simulink model "Commande_1_ModeGlissant"  (R2015a)
settings: Solver=ode45  StartTime=0.0  StopTime=5  RelTol=1e-3
undefined symbols (not defined in the file or in its folder): sfun3d
(part 1 of 2)
settings Model: Creator=user  LastModifiedBy=user

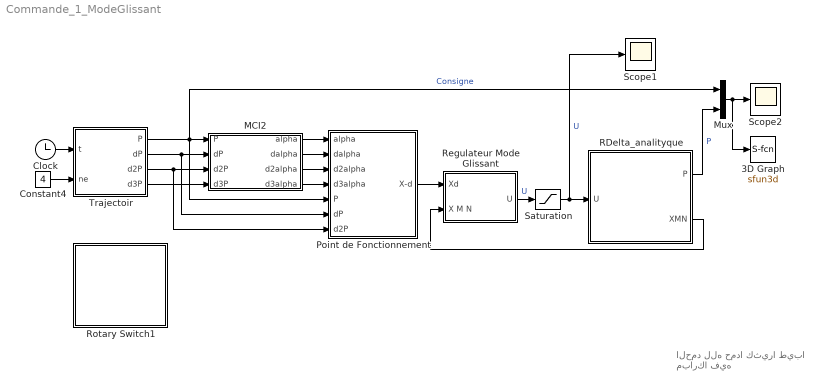
== system Commande_1_ModeGlissant ==
  note: الحمد لله حمدا كثيرا طيبا مباركا فيه
  3D Graph : S-Function  LoadFcn=sfun3d([],[],[],'LoadBlock')  StartFcn=sfun3d([],[],[],'Start')  StopFcn=sfun3d([],[],[],'Stop')  FunctionName=sfun3d  Parameters=ax,T,np,cp,gd,ls,mk  mask(3D Graph){np=2, ax=[-1 1 -1 1 -2 0]*0.3, cp=[3 2 1], gd=on, ls=-, mk=none, T=0.0001}
      mask prompts: np "Number of point (lines)"; ax "[xmin xmax  ymin ymax zmin zmax]"; cp "Camera position (use [0 0 1] for 2D XY view)"; gd "Grid (on|off)"; ls "LineStyle"; mk "Marker"; T "Sampling Time"
      mask help:
      | This block plots the position of several points in the XYZ space. The input contains the coordinates of all the points (x1,y1,z1,x2,y2,z2,...).
      | The number of points (lines), the XYZ ranges, camera position, grid, linestyle, marker and sampling time, can be set as mask parameters.
      settings: CopyFcn=sfun3d([],[],[],'CopyBlock')  DeleteFcn=sfun3d([],[],[],'DeleteBlock')  NameChangeFcn=sfun3d([],[],[],'NameChange')
      mask Help:
      | This block plots the position of several points in the XYZ space. The input contains the coordinates of all the points (x1,y1,z1,x2,y2,z2,...).
      | The number of points (lines), the XYZ ranges, camera position, grid, linestyle, marker and sampling time, can be set as mask parameters.
      mask TypeOptions ls: - | -- | : | -. | none
      mask TypeOptions mk: none | . | + | o | * | x | square | diamond | v | ^ | > | < | pentagram | hexagram
      mask Display: plot([.05 .95 .95 .05 .05],[.45 .45 .95 .95 .45], 0.5+cos(0:0.1:2*pi)*0.3,0.7+sin(0:0.1:2*pi)*0.2)
  Clock : Clock
  Constant4 : Constant  Value=4
  MCI2 : MATLAB Function  TreatAsAtomicUnit=on
  Mux : Mux  Inputs=2
  Point de Fonctionnement : Subsystem
  RDelta_analityque : Subsystem
      mask Display:
      | image(imread('DeltaImage2.PNG'))
      | 
      | port_label('input',1,'U')
      | 
      | port_label('output',1,'P')
      | 
      | port_label('output',2,'XMN')
  Regulateur Mode Glissant : Subsystem
  Rotary Switch1 : Subsystem  DialogController=hmiCreateDDGDialog  IsWebBlock=on  mask(MathWorksWebBlock){webBlockId=84b08da5-f823-455a-b5c0-7d4cf8879998, webBlockType=discreteknob, ShowInLibBrowser=on, ShowInitialText=on, HMISrcModelName=Commande_1_ModeGlissant}
      mask prompts: webBlockId "WebBlock Id"; webBlockType "WebBlock Type"; HMISrcModelName "Source Model"
      mask Help: helpview([docroot '/mapfiles/simulink.map'], 'hmi_rotary_switch')
      mask Display:
      | model = bdroot(gcb);
      | if strcmp(get_param(model,'BlockDiagramType'), 'library')
      |     image([(matlabroot) '/toolbox/simulink/hmi/icons/DiscreteKnob.png']);
      | end
  Saturation : Saturate  UpperLimit=24  LowerLimit=-24
  Scope1 : Scope
      settings: YMax=4.5
  Scope2 : Scope
      settings: YMin=-0.325  YMax=0.225
  Trajectoir : MATLAB Function  TreatAsAtomicUnit=on
  wires:
  RDelta_analityque/1(P) -> Mux/2  "P"
  Trajectoir/1(P) -> Point de Fonctionnement/5(P), Mux/1, MCI2/1(P)  "Consigne"
  Trajectoir/2(dP) -> Point de Fonctionnement/6(dP), MCI2/2(dP)
  Trajectoir/3(d2P) -> Point de Fonctionnement/7(d2P), MCI2/3(d2P)
  MCI2/3(d2alpha) -> Point de Fonctionnement/3(d2alpha)
  MCI2/2(dalpha) -> Point de Fonctionnement/2(dalpha)
  Clock/1 -> Trajectoir/1(t)
  Constant4/1 -> Trajectoir/2(ne)
  MCI2/1(alpha) -> Point de Fonctionnement/1(alpha)
  MCI2/4(d3alpha) -> Point de Fonctionnement/4(d3alpha)
  Trajectoir/4(d3P) -> MCI2/4(d3P)
  Mux/1 -> Scope2/1, 3D Graph/1
  Point de Fonctionnement/1(X-d) -> Regulateur Mode Glissant/1(Xd)
  RDelta_analityque/2(XMN) -> Regulateur Mode Glissant/2(X M N)
  Saturation/1 -> Scope1/1, RDelta_analityque/1(U)  "U"
  Regulateur Mode Glissant/1(U) -> Saturation/1  "U"

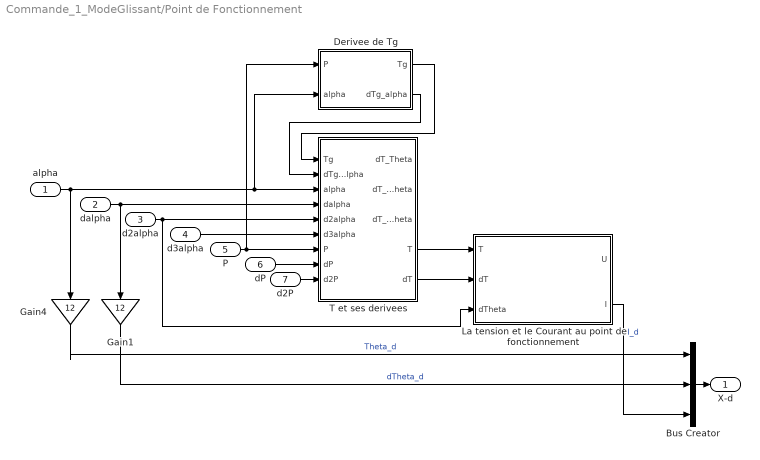
== system Commande_1_ModeGlissant/Point de Fonctionnement ==
  alpha : Inport
  dalpha : Inport  Port=2
  d2alpha : Inport  Port=3
  d3alpha : Inport  Port=4
  P : Inport  Port=5
  dP : Inport  Port=6
  d2P : Inport  Port=7
  Bus Creator : BusCreator  Inputs=3
  Derivee de Tg : Subsystem
  Gain1 : Gain  Gain=12
  Gain4 : Gain  Gain=12
  La tension et le Courant au point de fonctionnement : MATLAB Function  TreatAsAtomicUnit=on
  T et ses derivees : Subsystem
  X-d : Outport
  wires:
  alpha/1 -> Derivee de Tg/2(alpha), T et ses derivees/3(alpha), Gain4/1
  dalpha/1 -> Gain1/1, T et ses derivees/4(dalpha)
  P/1 -> Derivee de Tg/1(P), T et ses derivees/7(P)
  dP/1 -> T et ses derivees/8(dP)
  d2P/1 -> T et ses derivees/9(d2P)
  T et ses derivees/5(dT) -> La tension et le Courant au point de fonctionnement/2(dT)
  Derivee de Tg/2(dTg_alpha) -> T et ses derivees/2(dTg_alpha)
  Derivee de Tg/1(Tg) -> T et ses derivees/1(Tg)
  d3alpha/1 -> T et ses derivees/6(d3alpha)
  T et ses derivees/4(T) -> La tension et le Courant au point de fonctionnement/1(T)
  Bus Creator/1 -> X-d/1
  Gain4/1 -> Bus Creator/1  "Theta_d"
  Gain1/1 -> Bus Creator/2  "dTheta_d"
  d2alpha/1 -> La tension et le Courant au point de fonctionnement/3(dTheta), T et ses derivees/5(d2alpha)
  La tension et le Courant au point de fonctionnement/2(I) -> Bus Creator/3  "I_d"

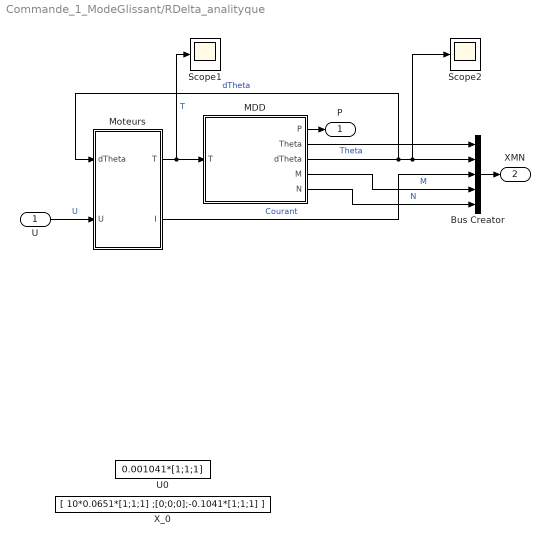
== system Commande_1_ModeGlissant/RDelta_analityque ==
  U : Inport
  Bus Creator : BusCreator  Inputs=5
  MDD : Subsystem
      mask Display:
      | image(imread('DeltaImage2.PNG'))
      | port_label('input',1,'T')
      | port_label('output',1,'P')
      | port_label('output',2,'Theta')
      | port_label('output',3,'dTheta')
      | port_label('output',4,'M')
      | port_label('output',5,'N')
  Moteurs : Subsystem
      mask Display:
      | image('image_motor.jpg')
      | port_label('output',1,'T')
      | port_label('output',2,'I')
      | port_label('input',1,'U')
      | port_label('input',2,'dTheta')
  Scope1 : Scope
      settings: YMin=-0.2  YMax=0.175  SaveName=ScopeData3
  Scope2 : Scope
      settings: YMin=0.774525  YMax=0.774531  SaveName=ScopeData7
  U0 : Constant  Value=0.001041*[1;1;1]
  X_0 : Constant  Value=[ 10*0.0651*[1;1;1] ;[0;0;0];-0.1041*[1;1;1] ]
  P : Outport
  XMN : Outport  Port=2
  wires:
  Moteurs/2(I) -> Bus Creator/3  "Courant"
  U/1 -> Moteurs/2(U)  "U"
  MDD/2(Theta) -> Bus Creator/1  "Theta"
  MDD/3(dTheta) -> Moteurs/1(dTheta), Bus Creator/2, Scope2/1  "dTheta"
  Moteurs/1(T) -> Scope1/1, MDD/1(T)  "T"
  MDD/1(P) -> P/1
  MDD/4(M) -> Bus Creator/4  "M"
  MDD/5(N) -> Bus Creator/5  "N"
  Bus Creator/1 -> XMN/1

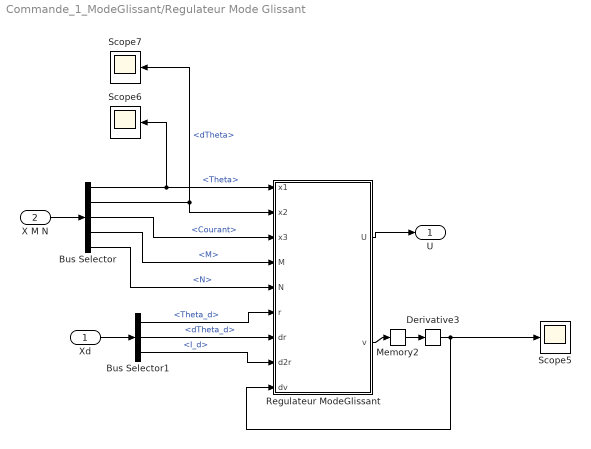
== system Commande_1_ModeGlissant/Regulateur Mode Glissant ==
  Xd : Inport
  X M N : Inport  Port=2
  Bus Selector : BusSelector  OutputSignals=Theta,dTheta,Courant,M,N
  Bus Selector1 : BusSelector  OutputSignals=Theta_d,dTheta_d,I_d
  Derivative3 : Derivative
  Memory2 : Memory  X0=[0;0;0]
  Regulateur ModeGlissant : MATLAB Function  TreatAsAtomicUnit=on
  Scope5 : Scope
      settings: YMin=-2000  YMax=18000  SaveName=ScopeData6
  Scope6 : Scope
      settings: YMin=-2000  YMax=18000  SaveName=ScopeData9
  Scope7 : Scope
      settings: YMin=-2000  YMax=18000  SaveName=ScopeData10
  U : Outport
  wires:
  Regulateur ModeGlissant/1(U) -> U/1
  Bus Selector/1 -> Scope6/1, Regulateur ModeGlissant/1(x1)  "<Theta>"
  Bus Selector/2 -> Scope7/1, Regulateur ModeGlissant/2(x2)  "<dTheta>"
  Bus Selector/3 -> Regulateur ModeGlissant/3(x3)  "<Courant>"
  Bus Selector/4 -> Regulateur ModeGlissant/4(M)  "<M>"
  Bus Selector/5 -> Regulateur ModeGlissant/5(N)  "<N>"
  X M N/1 -> Bus Selector/1
  Xd/1 -> Bus Selector1/1
  Regulateur ModeGlissant/2(v) -> Memory2/1
  Memory2/1 -> Derivative3/1
  Derivative3/1 -> Regulateur ModeGlissant/9(dv), Scope5/1
  Bus Selector1/1 -> Regulateur ModeGlissant/6(r)  "<Theta_d>"
  Bus Selector1/2 -> Regulateur ModeGlissant/7(dr)  "<dTheta_d>"
  Bus Selector1/3 -> Regulateur ModeGlissant/8(d2r)  "<I_d>"

== system Commande_1_ModeGlissant/Rotary Switch1 ==

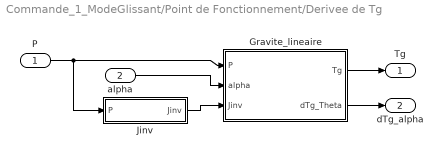
== system Commande_1_ModeGlissant/Point de Fonctionnement/Derivee de Tg ==
  P : Inport
  alpha : Inport  Port=2
  Gravite_lineaire : MATLAB Function  TreatAsAtomicUnit=on
  Jinv : MATLAB Function  TreatAsAtomicUnit=on
  Tg : Outport
  dTg_alpha : Outport  Port=2
  wires:
  P/1 -> Jinv/1(P), Gravite_lineaire/1(P)
  alpha/1 -> Gravite_lineaire/2(alpha)
  Jinv/1(Jinv) -> Gravite_lineaire/3(Jinv)
  Gravite_lineaire/2(dTg_Theta) -> dTg_alpha/1
  Gravite_lineaire/1(Tg) -> Tg/1

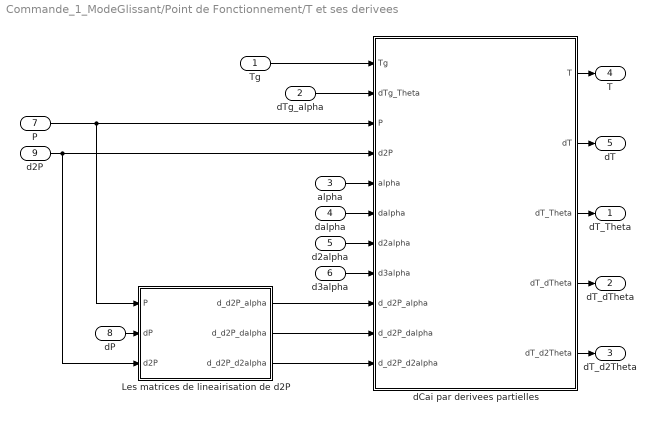
== system Commande_1_ModeGlissant/Point de Fonctionnement/T et ses derivees ==
  Tg : Inport
  dTg_alpha : Inport  Port=2
  alpha : Inport  Port=3
  dalpha : Inport  Port=4
  d2alpha : Inport  Port=5
  d3alpha : Inport  Port=6
  P : Inport  Port=7
  dP : Inport  Port=8
  d2P : Inport  Port=9
  "Les matrices de lineairisation de d2P  " : MATLAB Function  TreatAsAtomicUnit=on
  "dCai par derivees partielles " : MATLAB Function  TreatAsAtomicUnit=on
  dT_Theta : Outport
  dT_dTheta : Outport  Port=2
  dT_d2Theta : Outport  Port=3
  T : Outport  Port=4
  dT : Outport  Port=5
  wires:
  "Les matrices de lineairisation de d2P  "/2(d_d2P_dalpha) -> "dCai par derivees partielles "/10(d_d2P_dalpha)
  "Les matrices de lineairisation de d2P  "/3(d_d2P_d2alpha) -> "dCai par derivees partielles "/11(d_d2P_d2alpha)
  "Les matrices de lineairisation de d2P  "/1(d_d2P_alpha) -> "dCai par derivees partielles "/9(d_d2P_alpha)
  P/1 -> "Les matrices de lineairisation de d2P  "/1(P), "dCai par derivees partielles "/3(P)
  d2P/1 -> "Les matrices de lineairisation de d2P  "/3(d2P), "dCai par derivees partielles "/4(d2P)
  alpha/1 -> "dCai par derivees partielles "/5(alpha)
  dalpha/1 -> "dCai par derivees partielles "/6(dalpha)
  d2alpha/1 -> "dCai par derivees partielles "/7(d2alpha)
  dP/1 -> "Les matrices de lineairisation de d2P  "/2(dP)
  "dCai par derivees partielles "/3(dT_Theta) -> dT_Theta/1
  "dCai par derivees partielles "/4(dT_dTheta) -> dT_dTheta/1
  "dCai par derivees partielles "/5(dT_d2Theta) -> dT_d2Theta/1
  dTg_alpha/1 -> "dCai par derivees partielles "/2(dTg_Theta)
  Tg/1 -> "dCai par derivees partielles "/1(Tg)
  d3alpha/1 -> "dCai par derivees partielles "/8(d3alpha)
  "dCai par derivees partielles "/1(T) -> T/1
  "dCai par derivees partielles "/2(dT) -> dT/1

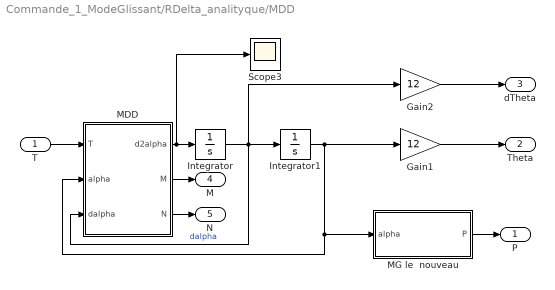
== system Commande_1_ModeGlissant/RDelta_analityque/MDD ==
  T : Inport
  Gain1 : Gain  Gain=12
  Gain2 : Gain  Gain=12
  Integrator : Integrator  InitialCondition=[0;0;0]
  Integrator1 : Integrator  InitialCondition=0.0651*[1;1;1]
  MDD : Subsystem
  MG le  nouveau : MATLAB Function  TreatAsAtomicUnit=on
  Scope3 : Scope
      settings: TimeRange=2.077341948455237  YMin=0.00075  YMax=0.00275  SaveName=ScopeData2
  P : Outport
  Theta : Outport  Port=2
  dTheta : Outport  Port=3
  M : Outport  Port=4
  N : Outport  Port=5
  wires:
  MDD/1(d2alpha) -> Scope3/1, Integrator/1
  Integrator/1 -> Gain2/1, MDD/3(dalpha), Integrator1/1  "dalpha"
  Integrator1/1 -> MG le  nouveau/1(alpha), MDD/2(alpha), Gain1/1
  T/1 -> MDD/1(T)
  MG le  nouveau/1(P) -> P/1
  Gain1/1 -> Theta/1
  Gain2/1 -> dTheta/1
  MDD/2(M) -> M/1
  MDD/3(N) -> N/1

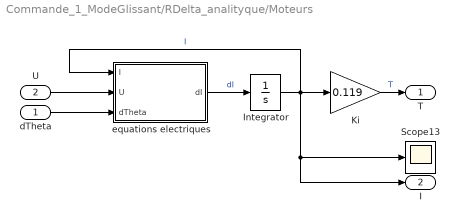
== system Commande_1_ModeGlissant/RDelta_analityque/Moteurs ==
  dTheta : Inport
  U : Inport  Port=2
  Integrator : Integrator  InitialCondition=-0.105*[1;1;1]
  Ki : Gain  Gain=0.119
  Scope13 : Scope
      settings: TimeRange=0.507510643892459  YMin=-1000  YMax=1000  SaveName=ScopeData24
  equations electriques : MATLAB Function  TreatAsAtomicUnit=on
  T : Outport
  I : Outport  Port=2
  wires:
  U/1 -> equations electriques/2(U)
  Integrator/1 -> Scope13/1, I/1, Ki/1, equations electriques/1(I)  "I"
  equations electriques/1(dI) -> Integrator/1  "dI"
  dTheta/1 -> equations electriques/3(dTheta)
  Ki/1 -> T/1  "T"

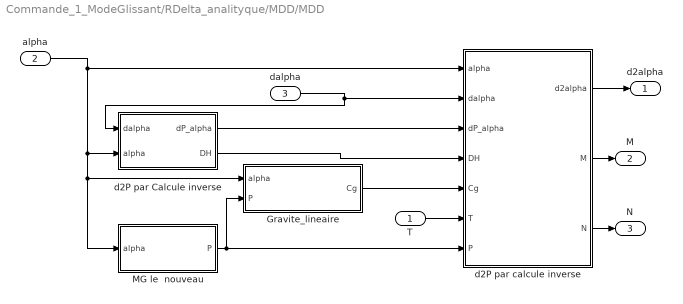
== system Commande_1_ModeGlissant/RDelta_analityque/MDD/MDD ==
  T : Inport
  alpha : Inport  Port=2
  dalpha : Inport  Port=3
  Gravite_lineaire : MATLAB Function  TreatAsAtomicUnit=on
  MG le  nouveau : MATLAB Function  TreatAsAtomicUnit=on
  "d2P par Calcule inverse " : Subsystem
  d2P par calcule inverse : MATLAB Function  TreatAsAtomicUnit=on
  d2alpha : Outport
  M : Outport  Port=2
  N : Outport  Port=3
  wires:
  d2P par calcule inverse/1(d2alpha) -> d2alpha/1
  "d2P par Calcule inverse "/1(dP_alpha) -> d2P par calcule inverse/3(dP_alpha)
  "d2P par Calcule inverse "/2(DH) -> d2P par calcule inverse/4(DH)
  MG le  nouveau/1(P) -> Gravite_lineaire/2(P), d2P par calcule inverse/7(P)
  dalpha/1 -> "d2P par Calcule inverse "/1(dalpha), d2P par calcule inverse/2(dalpha)
  alpha/1 -> MG le  nouveau/1(alpha), Gravite_lineaire/1(alpha), "d2P par Calcule inverse "/2(alpha), d2P par calcule inverse/1(alpha)
  Gravite_lineaire/1(Cg) -> d2P par calcule inverse/5(Cg)
  T/1 -> d2P par calcule inverse/6(T)
  d2P par calcule inverse/2(M) -> M/1
  d2P par calcule inverse/3(N) -> N/1

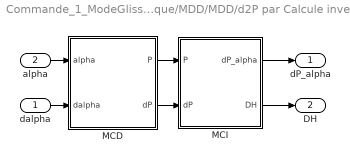
== system Commande_1_ModeGlissant/RDelta_analityque/MDD/MDD/d2P par Calcule inverse  ==
  dalpha : Inport
  alpha : Inport  Port=2
  MCD : MATLAB Function  TreatAsAtomicUnit=on
  MCI : MATLAB Function  TreatAsAtomicUnit=on
  dP_alpha : Outport
  DH : Outport  Port=2
  wires:
  MCD/2(dP) -> MCI/2(dP)
  MCD/1(P) -> MCI/1(P)
  alpha/1 -> MCD/1(alpha)
  dalpha/1 -> MCD/2(dalpha)
  MCI/1(dP_alpha) -> dP_alpha/1
  MCI/2(DH) -> DH/1

== matlab function Commande_1_ModeGlissant/RDelta_analityque/MDD/MDD/MG le  nouveau ==
  data: alpha input; P output
function P =MGD(alpha)


alpha1=alpha(1) ;alpha2=alpha(2) ; alpha3=alpha(3) ;

%les constantes
l1 = 0.19992; 
l2 = 0.334; 
r = 0.126; 
phi2 = 2*pi/3;
phi3 = 4*pi/3;

%% Les points :
C1=[r+l1*cos(alpha1) ; 0 ; -l1*sin(alpha1) ]; 
C2=[(r+l1*cos(alpha2))*cos(phi2) ; (r+l1*cos(alpha2))*sin(phi2) ; -l1*sin(alpha2) ]; 
C3=[(r+l1*cos(alpha3))*cos(phi3) ; (r+l1*cos(alpha3))*sin(phi3) ; -l1*sin(alpha3) ]; 

%% Les vecteurs du triangle C1C2C3 et ses distances
C1C2= C2-C1 ; C2C3 =C3-C2 ; C3C1= C1-C3 ;
a=sqrt(C1C2'*C1C2) ; b=sqrt(C2C3'*C2C3)  ; c=sqrt(C3C1'*C3C1)  ;
 p= a+b+c ; % Le perimetre de C1C2C3
 R = a*b*c/sqrt(p*(p-2*a)*(p-2*b)*(p-2*c)) ;

 %% Calcule du point L 
 % Les vecteurs u et n:
 v1=C1C2/a ;
 n=cross(C3C1,C1C2)*2*R/(a*b*c) ;
 TL = sqrt(R^2-a^2/4) ;
 OL=(C1+C2)/2+TL*sign(-a*a+c*c+b*b)*cross(n,v1);
 %% Calcule du point E :
P=OL-sqrt(l2^2-R^2)*n ;

== matlab function Commande_1_ModeGlissant/MCI2 ==
  data: P input; dP input; d2P input; d3P input; alpha output; dalpha output; d2alpha output; d3alpha output
    function [alpha, dalpha,d2alpha,d3alpha]= fcn(P,dP,d2P,d3P)

    l1 = 0.19992; 
    l2 = 0.334; 
    r = 0.126; 
    phi2 = 2*pi/3;
    phi3 = 4*pi/3;

    %% Expression de P dans Ri
    % l'expression P1 dP1 et d2P1 ne se changent pas
    A2=[cos(phi2) sin(phi2) 0
        -sin(phi2) cos(phi2) 0
        0            0      1 ]; 
    A3=[cos(phi3) sin(phi3) 0
        -sin(phi3) cos(phi3) 0
        0            0      1 ];
     P2=A2*P; dP2=A2*dP; d2P2=A2*d2P; d3P2=A2*d3P;
     P3=A3*P ; dP3=A3*dP ; d2P3=A3*d2P ; d3P3=A3*d3P;
        
    x1=P(1); y1=P(2) ; z1=P(3) ; 
    x2=P2(1); y2=P2(2) ; z2=P2(3) ;
    x3=P3(1); y3=P3(2) ; z3=P3(3) ;
    % Notation de dP :
    dx1=dP(1); dy1=dP(2) ; dz1=dP(3) ; 
    dx2=dP2(1); dy2=dP2(2) ; dz2=dP2(3) ; 
    dx3=dP3(1); dy3=dP3(2) ; dz3=dP3(3) ; 
    % Notation de d2P :
    d2x1=d2P(1); d2y1=d2P(2) ; d2z1=d2P(3) ;
    d2x2=d2P2(1); d2y2=d2P2(2) ; d2z2=d2P2(3) ;
    d2x3=d2P3(1); d2y3=d2P3(2) ; d2z3=d2P3(3) ;
    % Notation de d3P :
    d3x1=d3P(1); d3y1=d3P(2) ; d3z1=d3P(3) ;
    d3x2=d3P2(1); d3y2=d3P2(2) ; d3z2=d3P2(3) ;
    d3x3=d3P3(1); d3y3=d3P3(2) ; d3z3=d3P3(3) ;
    % L'expression de dP dans Ri :
      

    %% Parametres du Triangle AiCiBi :
    % Triangle 1 :
    AB1=sqrt(z1^2+(x1-r)^2);
    e1=sqrt(l2^2-y1^2); 
    AB2=sqrt(z2^2+(x2-r)^2);
    e2=sqrt(l2^2-y2^2);
    AB3=sqrt(z3^2+(x3-r)^2);
    e3=sqrt(l2^2-y3^2);

    %% calcul de alpha1
    beta1=atan2(-z1,x1-r);
    delta1=acos((AB1^2 + l1^2 - e1^2)/(2*l1*AB1));
    alpha1=beta1-delta1; 


    %% calcul de alpha2
    beta2=atan2(-z2,x2-r);
    delta2=acos((AB2^2 + l1^2 - e2^2)/(2*l1*AB2));
    alpha2=beta2-delta2; 


    %% calcul de alpha3
    beta3=atan2(-z3,x3-r);
    delta3=acos((AB3^2 + l1^2 - e3^2)/(2*l1*AB3));
    alpha3=beta3-delta3; 

% Tranformation au Deg
alpha=[alpha1;alpha2;alpha3]; % first solution


%% =================== Calcule de dalpha_i ====================================

% ---------------------------- Calcul de dAlpha1 ----------------------
% Calcule de dDelta1 :
BH1 = AB1-l1*cos(delta1);
D1=l1*AB1*sin(delta1) ;
dDelta1X = -BH1*(x1-r)/AB1/D1 ; 
dDelta1Y = -y1/D1 ; 
dDelta1Z = -BH1*z1/AB1/D1 ; 
Gdelta1=  [ dDelta1X , dDelta1Y , dDelta1Z] ;
dDelta1 = Gdelta1*dP ;
% Calcule de dBeta1 :
dBeta1Z=-(x1-r)/AB1^2 ; dBeta1X=z1/AB1^2 ;
Gbeta1=[ dBeta1X ,  0 , dBeta1Z] ;
dBeta1 = Gbeta1*dP;
% Calcule de dAlpha1 :
Galpha1=Gbeta1-Gdelta1 ;
dAlpha1 = Galpha1*dP ;

% ---------------------------- Calcul de dAlpha2 ----------------------
% Calcule de dDelta2 :
BH2 = AB2-l1*cos(delta2);
D2=l1*AB2*sin(delta2) ;
dDelta2X = -BH2*(x2-r)/AB2/D2 ; 
dDelta2Y = -y2/D2 ; 
dDelta2Z = -BH2*z2/AB2/D2 ; 
Gdelta2=  [ dDelta2X , dDelta2Y , dDelta2Z] ;
dDelta2 = Gdelta2*dP2 ;
% Calcule de dBeta2 :
dBeta2Z=-(x2-r)/AB2^2 ; dBeta2X=z2/AB2^2 ;
Gbeta2=[ dBeta2X ,  0 , dBeta2Z] ;
dBeta2 = Gbeta2*dP2;
% Calcule de dAlpha2 :
Galpha2=Gbeta2-Gdelta2 ;
dAlpha2 = Galpha2*dP2 ;

% ---------------------------- Calcul de dAlpha3 ----------------------
% Calcule de dDelta2 :
BH3 = AB3-l1*cos(delta3);
D3=l1*AB3*sin(delta3) ;
dDelta3X = -BH3*(x3-r)/AB3/D3 ; 
dDelta3Y = -y3/D3 ; 
dDelta3Z = -BH3*z3/AB3/D3 ; 
Gdelta3=  [ dDelta3X , dDelta3Y , dDelta3Z] ;
dDelta3 = Gdelta3*dP3 ;
% Calcule de dBeta3:
dBeta3Z=-(x3-r)/AB3^2 ; dBeta2X=z3/AB3^2 ;
Gbeta3=[ dBeta2X ,  0 , dBeta3Z] ;
dBeta3 = Gbeta3*dP3;
% Calcule de dAlpha3 :
Galpha3=Gbeta3-Gdelta3 ;
dAlpha3 = Galpha3*dP3 ;

dalpha=[ dAlpha1 ; dAlpha2 ; dAlpha3 ];

%% ===================== Calcule de d2alpha_i =================================
 
% ---------------------------- Calcul de d2Alpha1 ----------------------
% Calcule de d2Gama1 :
CH1=l1*sin(delta1);
AH1=l1*cos(delta1) ;
d2Delta1XX = -BH1*(x1-r)^2/(AB1^3*D1)*( AH1*e1^2/(BH1*CH1^2) + (AB1/(x1-r))^2 - 2 ) ;
d2Delta1YY = - (1+y1^2*AH1*AB1/D1^2 )  /D1;
d2Delta1ZZ  = -BH1*z1^2/(AB1^3*D1)*( AH1*e1^2/(BH1*CH1^2) + (AB1/z1)^2 -2 ) ;
d2Delta1XY = y1*(x1-r)*(CH1^2-AH1*BH1)/D1^3 ;
d2Delta1XZ = -BH1*(x1-r)*z1/(AB1^3*D1)*( AH1*e1^2/(BH1*CH1^2) - 2 ) ;
d2Delta1YZ = y1*z1*(CH1^2-AH1*BH1)/D1^3 ; 
Hdelta1=[ d2Delta1XX,d2Delta1XY,d2Delta1XZ ; d2Delta1XY, d2Delta1YY,d2Delta1YZ ;d2Delta1XZ , d2Delta1YZ,d2Delta1ZZ] ;
d2Delta1=dP'*Hdelta1*dP +  Gdelta1*d2P ; 
%Calcule de dBeta 1:
d2Beta1XX=-2*(x1-r)*z1/AB1^4 ; d2Beta1ZZ=-d2Beta1XX ; d2Beta1XZ = ((x1-r)^2-z1^2)/AB1^4 ;
Hbeta1= [d2Beta1XX , 0, d2Beta1XZ ; 0, 0, 0 ; d2Beta1XZ , 0 , d2Beta1ZZ ] ;
d2Beta1=dP'*Hbeta1*dP + Gbeta1*d2P;
%Calcule de dAlpha1 :
Halpha1= Hbeta1 - Hdelta1; 
d2Alpha1=dP'*Halpha1*dP + Galpha1*d2P;

% ---------------------------- Calcul de d2Alpha2 ----------------------
% Calcule de d2Gama1 :
CH2=l1*sin(delta2);
AH2=l1*cos(delta2) ;
d2Delta2XX = -BH2*(x2-r)^2/(AB2^3*D2)*( AH2*e2^2/(BH2*CH2^2) + (AB2/(x2-r))^2 - 2 ) ;
d2Delta2YY = - (1+y2^2*AH2*AB2/D2^2 )  /D2;
d2Delta2ZZ  = -BH2*z2^2/(AB2^3*D2)*( AH2*e2^2/(BH2*CH2^2) + (AB2/z2)^2 -2 ) ;
d2Delta2XY = y2*(x2-r)*(CH2^2-AH2*BH2)/D2^3 ;
d2Delta2XZ = -BH2*(x2-r)*z2/(AB2^3*D2)*( AH2*e2^2/(BH2*CH2^2) - 2 ) ;
d2Delta2YZ = y2*z2*(CH2^2-AH2*BH2)/D2^3 ; 
Hdelta2=[ d2Delta2XX,d2Delta2XY,d2Delta2XZ ; d2Delta2XY, d2Delta2YY,d2Delta2YZ ;d2Delta2XZ , d2Delta2YZ,d2Delta2ZZ] ;
d2Delta1=dP2'*Hdelta2*dP2 +  Gdelta2*d2P2 ; 
%Calcule de dBeta2:
d2Beta2XX=-2*(x2-r)*z2/AB2^4 ; d2Beta2ZZ=-d2Beta2XX ; d2Beta2XZ = ((x2-r)^2-z2^2)/AB2^4 ;
Hbeta2= [d2Beta2XX , 0, d2Beta2XZ ; 0, 0, 0 ; d2Beta2XZ , 0 , d2Beta2ZZ ] ;
d2Beta2=dP2'*Hbeta2*dP2 + Gbeta2*d2P2;
%Calcule de dAlpha2 :
Halpha2= Hbeta2 - Hdelta2; 
d2Alpha2=dP2'*Halpha2*dP2 + Galpha2*d2P2;

% ---------------------------- Calcul de d2Alpha3 ----------------------
% Calcule de d2Gama3 :
CH3=l1*sin(delta3);
AH3=l1*cos(delta3) ;
d2Delta3XX = -BH3*(x3-r)^2/(AB3^3*D3)*( AH3*e3^2/(BH3*CH3^2) + (AB3/(x3-r))^2 - 2 ) ;
d2Delta3YY = - (1+y3^2*AH3*AB3/D3^2 )  /D3;
d2Delta3ZZ  = -BH3*z3^2/(AB3^3*D3)*( AH3*e3^2/(BH3*CH3^2) + (AB3/z3)^2 -2 ) ;
d2Delta3XY = y3*(x3-r)*(CH3^2-AH3*BH3)/D3^3 ;
d2Delta3XZ = -BH3*(x3-r)*z3/(AB3^3*D3)*( AH3*e3^2/(BH3*CH3^2) - 2 ) ;
d2Delta3YZ = y3*z3*(CH3^2-AH3*BH3)/D3^3 ; 
Hdelta3=[ d2Delta3XX,d2Delta3XY,d2Delta3XZ ; d2Delta3XY, d2Delta3YY,d2Delta3YZ ;d2Delta3XZ , d2Delta3YZ,d2Delta3ZZ] ;
d2Delta3=dP3'*Hdelta3*dP3 +  Gdelta3*d2P3 ; 
%Calcule de dBeta3:
d2Beta3XX=-2*(x3-r)*z3/AB3^4 ; d2Beta3ZZ=-d2Beta3XX ; d2Beta3XZ = ((x3-r)^2-z3^2)/AB3^4 ;
Hbeta3= [d2Beta3XX , 0, d2Beta3XZ ; 0, 0, 0 ; d2Beta3XZ , 0 , d2Beta3ZZ ] ;
d2Beta2=dP3'*Hbeta3*dP3 + Gbeta3*d2P3;
%Calcule de dAlpha3 :
Halpha3= Hbeta3 - Hdelta3; 
d2Alpha3=dP3'*Halpha3*dP3 + Galpha3*d2P3;

d2alpha=[d2Alpha1 ; d2Alpha2 ; d2Alpha3];

%%  Autres formule pour calculer d2Delta :
% % ---------------------------- Calcul de d2Alpha1 ----------------------
% % Calcule de d2Delta1 :
% dAB1 = ( z1*dz1 + (x1-r)*dx1 )/AB1 ;
% d2AB1 = (dz1^2 + z1*d2z1 + dx1^2 + (x1-r)*d2x1 -dAB1^2 )/AB1 ;
% de1=(-y1*dy1)/e1 ;
% d2e1 = -(dy1^2 + y1*d2y1 + de1^2)/e1 ;
% d2Delta1=( dAB1^2 + AB1*d2AB1 - de1^2 - e1*d2e1 -l1*(d2AB1*cos(delta1)-2*dAB1*sin(delta1)*dDelta1 - AB1*cos(delta1)*dDelta1^2) )  /(-l1*AB1*sin(delta1));


%% ==================== Caclcule de d3Alpahi ==================

%% ------------------------------ 1)  Calcule de d3Alpha1 -----------------------------
% Calcule de d3Delta1 :
% Parametres (1er derivees):
DH1=CH1^2-AH1*BH1 ;
dAB1X=(x1-r)/AB1 ; dAB1Z = z1/AB1 ; 
dD1X=(x1-r)*DH1/D1 ; dD1Z= z1*DH1/D1; dD1Y=-y1*AH1/CH1 ;
dD1=dD1Z*dz1 ;%dD1X*dx1+ dD1Y*dy1 +
dAH1X=(x1-r)*BH1/AB1^2 ; dAH1Z = z1*BH1/AB1^2  ; dAH1Y=y1/AB1 ;
dBH1X=(x1-r)*AH1/AB1^2 ; dBH1Z = z1*AH1/AB1^2  ; dBH1Y=-y1/AB1 ;
dCH1X= -(x1-r)*AH1*BH1/CH1/AB1^2 ; dCH1Z=-z1*AH1*BH1/CH1/AB1^2 ; 
dCH1Y= -y1*AH1/D1 ;
dCH1=dCH1Z*dz1 ;
% Parametres (2eme derivees partielles):
% d2D1
d2D1XX=(DH1-(x1-r)^2-(dD1X)^2)/D1 ;
d2D1ZZ=(DH1-z1^2-(dD1Z)^2)/D1 ;
d2D1YY= -AH1/CH1-y1^2/D1*(1+(AH1/CH1)^2);
d2D1XZ = -(z1*(x1-r) + dD1X*dD1Z)/D1 ;
d2D1XY=-(y1*(x1-r) + dD1X*dD1Y)/D1  ;
d2D1ZY=-(z1*y1 + dD1Y*dD1Z)/D1 ;
% d2AB1
d2AB1XX = 1/AB1 - (x1-r)*dAB1X/AB1^2 ;
d2AB1ZZ= 1/AB1 - z1*dAB1Z/AB1^2 ;
d2AB1XZ=-z1*(x1-r)/AB1^3;
%d2BH1
d2BH1ZZ=dBH1Z*(dAH1Z/AH1 +1/z1 - 2*dAB1Z/AB1) ;
d2BH1XX=dBH1X*(dAH1X/AH1 +1/(x1-r) - 2*dAB1X/AB1) ;
d2BH1XZ=z1*(x1-r)*(BH1-2*AH1)/AB1^4 ;

%------------------- les derivees partielles  d3Delta1_
d3Delta1ZZZ = d2Delta1ZZ*(dBH1Z/BH1+1/z1-dAB1Z/AB1-dD1Z/D1) + dDelta1Z*(-(dBH1Z/BH1)^2-1/z1^2+(dAB1Z/AB1)^2+(dD1Z/D1)^2 + d2BH1ZZ/BH1 - d2AB1ZZ/AB1 -d2D1ZZ/D1);
d3Delta1XXX = d2Delta1XX*(dBH1X/BH1+1/(x1-r)-dAB1X/AB1-dD1X/D1) + dDelta1X*(-(dBH1X/BH1)^2-1/(x1-r)^2+(dAB1X/AB1)^2+(dD1X/D1)^2 + d2BH1XX/BH1 - d2AB1XX/AB1 -d2D1XX/D1);
d3Delta1YYY= dD1Y/D1^2 + D1^2\(dD1Y + y1*d2D1YY-2*(dD1Y)^2*y1/D1);
d3Delta1XZZ= d2Delta1XZ*(dBH1Z/BH1+1/z1-dAB1Z/AB1-dD1Z/D1)+dDelta1Z*(-dBH1X*dBH1Z/BH1^2 + dAB1Z*dAB1X/AB1^2 + dD1Z*dD1X/D1^2 + d2BH1XZ/BH1 - d2AB1XZ/AB1 -d2D1XZ/D1) ;
d3Delta1XXZ= d2Delta1XZ*(dBH1X/BH1+1/(x1-r)-dAB1X/AB1-dD1X/D1)+dDelta1X*(-dBH1X*dBH1Z/BH1^2 + dAB1Z*dAB1X/AB1^2 + dD1Z*dD1X/D1^2 + d2BH1XZ/BH1 - d2AB1XZ/AB1 -d2D1XZ/D1) ;
d3Delta1XYY=(x1-r)/D1^3*(DH1-y1^2-3*y1*DH1*dD1Y/D1);
d3Delta1XXY=y1/D1^3*(DH1-(x1-r)^2*(1+3*(DH1/D1)^2));
d3Delta1YYZ=z1/D1^3*(DH1-y1^2-3*y1*DH1*dD1Y/D1);
d3Delta1YZZ=y1/D1^3*(DH1-z1^2*(1+3*(DH1/D1)^2));
d3Delta1XYZ=-(x1-r)*y1*z1/D1^3*(1+3*(DH1/D1)^2);
dHdelta1X=[ d3Delta1XXX,d3Delta1XXY,d3Delta1XXZ ; d3Delta1XXY, d3Delta1XYY,d3Delta1XYZ ;d3Delta1XXZ , d3Delta1XYZ,d3Delta1XZZ] ;
dHdelta1Y=[ d3Delta1XXY,d3Delta1XYY,d3Delta1XYZ ; d3Delta1XYY, d3Delta1YYY,d3Delta1YYZ ;d3Delta1XYZ , d3Delta1YYZ,d3Delta1YZZ] ;
dHdelta1Z=[ d3Delta1XXZ,d3Delta1XYZ,d3Delta1XZZ ; d3Delta1XYZ, d3Delta1YYZ,d3Delta1YZZ ;d3Delta1XZZ , d3Delta1YZZ,d3Delta1ZZZ] ;
d3Delta1= 3*dP'*Hdelta1*d2P + Gdelta1*d3P + dP'*[dHdelta1X*dP,dHdelta1Y*dP , dHdelta1Z*dP]*dP ;
%---------------  les derivees partielles  d3Beta1_
d3Beta1XXX=-2*z1/AB1^4*(1-4*((x1-r)/AB1)^2) ; 
d3Beta1ZZZ=2*(x1-r)/AB1^4*(1-4*(z1/AB1)^2) ; 
d3Beta1XZZ=-d3Beta1XXX;d3Beta1XXZ=-d3Beta1ZZZ ;
dHbeta1X=[d3Beta1XXX , 0 ,d3Beta1XXZ ; 0,0,0;d3Beta1XXZ , 0 , d3Beta1XZZ];
dHbeta1Z=[d3Beta1XXZ , 0 ,d3Beta1XZZ ; 0,0,0;d3Beta1XZZ , 0 , d3Beta1ZZZ];
dHbeta1Y= zeros(3) ;
d3Beta1=3*dP'*Hbeta1*d2P + Gbeta1*d3P + dP'*[dHbeta1X*dP,dHbeta1Y*dP, dHbeta1Z*dP]*dP ;
% En fin :
dHalpha1X=dHbeta1X-dHdelta1X ;
dHalpha1Y=dHbeta1Y-dHdelta1Y ;
dHalpha1Z=dHbeta1Z-dHdelta1Z ;
d3Alpha1=3*dP'*Halpha1*d2P + Galpha1*d3P + dP'*[dHalpha1X*dP,dHalpha1Y*dP, dHalpha1Z*dP]*dP ;
%% -------------------------------2) Calcule de d3Alpha2 -----------------------------
% Calcule de d3Delta2 :
% Parametres (1er derivees):
DH2=CH2^2-AH2*BH2 ;
dAB2X=(x2-r)/AB2 ; dAB2Z = z2/AB2 ; 
dD2X=(x2-r)*DH2/D2 ; dD2Z= z2*DH2/D2; dD2Y=-y2*AH2/CH2 ;
dAH2X=(x2-r)*BH2/AB2^2 ; dAH2Z = z2*BH2/AB2^2  ; dAH2Y=y2/AB2 ;
dBH2X=(x2-r)*AH2/AB2^2 ; dBH2Z = z2*AH2/AB2^2  ; dBH2Y=-y2/AB2 ;
dCH2X= -(x2-r)*AH2*BH2/CH2/AB2^2 ; dCH2Z=-z2*AH2*BH2/CH2/AB2^2 ; 
dCH2Y= -y2*AH2/D2 ;
dCH2=dCH2Z*dz2 ;
% Parametres (2eme derivees partielles):
% d2D2
d2D2XX=(DH2-(x2-r)^2-(dD2X)^2)/D2 ;
d2D2ZZ=(DH2-z2^2-(dD2Z)^2)/D2 ;
d2D2YY= -AH2/CH2-y2^2/D2*(1+(AH2/CH2)^2);
d2D2XZ = -(z2*(x2-r) + dD2X*dD2Z)/D2 ;
d2D2XY=-(y2*(x2-r) + dD2X*dD2Y)/D2  ;
d2D2ZY=-(z2*y2 + dD2Y*dD2Z)/D2 ;
% d2AB2
d2AB2XX = 1/AB2 - (x2-r)*dAB2X/AB2^2 ;
d2AB2ZZ= 1/AB2 - z2*dAB2Z/AB2^2 ;
d2AB2XZ=-z2*(x2-r)/AB2^3;
%d2BH2
d2BH2ZZ=dBH2Z*(dAH2Z/AH2 +1/z2 - 2*dAB2Z/AB2) ;
d2BH2XX=dBH2X*(dAH2X/AH2 +1/(x2-r) - 2*dAB2X/AB2) ;
d2BH2XZ=z2*(x2-r)*(BH2-2*AH2)/AB2^4 ;

%------------- les derivees partielles  d3Delta1_
d3Delta2ZZZ = d2Delta2ZZ*(dBH2Z/BH2+1/z2-dAB2Z/AB2-dD2Z/D2) + dDelta2Z*(-(dBH2Z/BH2)^2-1/z2^2+(dAB2Z/AB2)^2+(dD2Z/D2)^2 + d2BH2ZZ/BH2 - d2AB2ZZ/AB2 -d2D2ZZ/D2);
d3Delta2XXX = d2Delta2XX*(dBH2X/BH2+1/(x2-r)-dAB2X/AB2-dD2X/D2) + dDelta2X*(-(dBH2X/BH2)^2-1/(x2-r)^2+(dAB2X/AB2)^2+(dD2X/D2)^2 + d2BH2XX/BH2 - d2AB2XX/AB2 -d2D2XX/D2);
d3Delta2YYY= dD2Y/D2^2 + D2^2\(dD2Y + y2*d2D2YY-2*(dD2Y)^2*y2/D2);
d3Delta2XZZ= d2Delta2XZ*(dBH2Z/BH2+1/z2-dAB2Z/AB2-dD2Z/D2)+dDelta2Z*(-dBH2X*dBH2Z/BH2^2 + dAB2Z*dAB2X/AB2^2 + dD2Z*dD2X/D2^2 + d2BH2XZ/BH2 - d2AB2XZ/AB2 -d2D2XZ/D2) ;
d3Delta2XXZ= d2Delta2XZ*(dBH2X/BH2+1/(x2-r)-dAB2X/AB2-dD2X/D2)+dDelta2X*(-dBH2X*dBH2Z/BH2^2 + dAB2Z*dAB2X/AB2^2 + dD2Z*dD2X/D2^2 + d2BH2XZ/BH2 - d2AB2XZ/AB2 -d2D2XZ/D2) ;
d3Delta2XYY=(x2-r)/D2^3*(DH2-y2^2-3*y2*DH2*dD2Y/D2);
d3Delta2XXY=y2/D2^3*(DH2-(x2-r)^2*(1+3*(DH2/D2)^2));
d3Delta2YYZ=z2/D2^3*(DH2-y2^2-3*y2*DH2*dD2Y/D2);
d3Delta2YZZ=y2/D2^3*(DH2-z2^2*(1+3*(DH2/D2)^2));
d3Delta2XYZ=-(x2-r)*y2*z2/D2^3*(1+3*(DH2/D2)^2);
dHdelta2X=[ d3Delta2XXX,d3Delta2XXY,d3Delta2XXZ ; d3Delta2XXY, d3Delta2XYY,d3Delta2XYZ ;d3Delta2XXZ , d3Delta2XYZ,d3Delta2XZZ] ;
dHdelta2Y=[ d3Delta2XXY,d3Delta2XYY,d3Delta2XYZ ; d3Delta2XYY, d3Delta2YYY,d3Delta2YYZ ;d3Delta2XYZ , d3Delta2YYZ,d3Delta2YZZ] ;
dHdelta2Z=[ d3Delta2XXZ,d3Delta2XYZ,d3Delta2XZZ ; d3Delta2XYZ, d3Delta2YYZ,d3Delta2YZZ ;d3Delta2XZZ , d3Delta2YZZ,d3Delta2ZZZ] ;
d3Delta1= 3*dP2'*Hdelta2*d2P2 + Gdelta2*d3P2 + dP2'*[dHdelta2X*dP2,dHdelta2Y*dP2 , dHdelta2Z*dP2]*dP2 ;
%%  les derivees partielles  d3Beta2_
d3Beta2XXX=-2*z2/AB2^4*(1-4*((x2-r)/AB2)^2) ; 
d3Beta2ZZZ=2*(x2-r)/AB2^4*(1-4*(z2/AB2)^2) ; 
d3Beta2XZZ=-d3Beta2XXX;d3Beta1XXZ=-d3Beta2ZZZ ;
dHbeta2X=[d3Beta2XXX , 0 ,d3Beta1XXZ ; 0,0,0;d3Beta1XXZ , 0 , d3Beta2XZZ];
dHbeta2Z=[d3Beta1XXZ , 0 ,d3Beta2XZZ ; 0,0,0;d3Beta2XZZ , 0 , d3Beta2ZZZ];
dHbeta2Y= zeros(3) ;
d3Beta2=3*dP2'*Hbeta2*d2P2 + Gbeta2*d3P2 + dP2'*[dHbeta2X*dP2,dHbeta2Y*dP2, dHbeta2Z*dP2]*dP2 ;
% En fin :
dHalpha2X=dHbeta2X-dHdelta2X ;
dHalpha2Y=dHbeta2Y-dHdelta2Y ;
dHalpha2Z=dHbeta2Z-dHdelta2Z ;
d3Alpha2=3*dP2'*Halpha2*d2P2 + Galpha2*d3P2 + dP2'*[dHalpha2X*dP2,dHalpha2Y*dP2, dHalpha2Z*dP2]*dP2 ;

%% -------------------------------3) Calcule de d3Alpha3 -----------------------------
% Calcule de d3Delta3 :
% Parametres (1er derivees):
DH3=CH3^2-AH3*BH3 ;
dAB3X=(x3-r)/AB3 ; dAB3Z = z3/AB3 ; 
dD3X=(x3-r)*DH3/D3 ; dD3Z= z3*DH3/D3; dD3Y=-y3*AH3/CH3 ;
dAH3X=(x3-r)*BH3/AB3^2 ; dAH3Z = z3*BH3/AB3^2  ; dAH3Y=y3/AB3 ;
dBH3X=(x3-r)*AH3/AB3^2 ; dBH3Z = z3*AH3/AB3^2  ; dBH3Y=-y3/AB3 ;
dCH3X= -(x3-r)*AH3*BH3/CH3/AB3^2 ; dCH3Z=-z3*AH3*BH3/CH3/AB3^2 ; 
dCH3Y= -y3*AH3/D3 ;
dCH3=dCH3Z*dz3 ;
% Parametres (2eme derivees partielles):
% d2D3
d2D3XX=(DH3-(x3-r)^2-(dD3X)^2)/D3 ;
d2D3ZZ=(DH3-z3^2-(dD3Z)^2)/D3 ;
d2D3YY= -AH3/CH3-y3^2/D3*(1+(AH3/CH3)^2);
d2D3XZ = -(z3*(x3-r) + dD3X*dD3Z)/D3 ;
d2D3XY=-(y3*(x3-r) + dD3X*dD3Y)/D3  ;
d2D3ZY=-(z3*y3 + dD3Y*dD3Z)/D3 ;
% d2AB3
d2AB3XX = 1/AB3 - (x3-r)*dAB3X/AB3^2 ;
d2AB3ZZ= 1/AB3 - z3*dAB3Z/AB3^2 ;
d2AB3XZ=-z3*(x3-r)/AB3^3;
%d2BH3
d2BH3ZZ=dBH3Z*(dAH3Z/AH3 +1/z3 - 2*dAB3Z/AB3) ;
d2BH3XX=dBH3X*(dAH3X/AH3 +1/(x3-r) - 2*dAB3X/AB3) ;
d2BH3XZ=z3*(x3-r)*(BH3-2*AH3)/AB3^4 ;


%%  les derivees partielles  d3Delta3_
d3Delta3ZZZ = d2Delta3ZZ*(dBH3Z/BH3+1/z3-dAB3Z/AB3-dD3Z/D3) + dDelta3Z*(-(dBH3Z/BH3)^2-1/z3^2+(dAB3Z/AB3)^2+(dD3Z/D3)^2 + d2BH3ZZ/BH3 - d2AB3ZZ/AB3 -d2D3ZZ/D3);
d3Delta3XXX = d2Delta3XX*(dBH3X/BH3+1/(x3-r)-dAB3X/AB3-dD3X/D3) + dDelta3X*(-(dBH3X/BH3)^2-1/(x3-r)^2+(dAB3X/AB3)^2+(dD3X/D3)^2 + d2BH3XX/BH3 - d2AB3XX/AB3 -d2D3XX/D3);
d3Delta3YYY= dD3Y/D3^2 + D3^2\(dD3Y + y3*d2D3YY-2*(dD3Y)^2*y3/D3);
d3Delta3XZZ= d2Delta3XZ*(dBH3Z/BH3+1/z3-dAB3Z/AB3-dD3Z/D3)+dDelta3Z*(-dBH3X*dBH3Z/BH3^2 + dAB3Z*dAB3X/AB3^2 + dD3Z*dD3X/D3^2 + d2BH3XZ/BH3 - d2AB3XZ/AB3 -d2D3XZ/D3) ;
d3Delta3XXZ= d2Delta3XZ*(dBH3X/BH3+1/(x3-r)-dAB3X/AB3-dD3X/D3)+dDelta3X*(-dBH3X*dBH3Z/BH3^2 + dAB3Z*dAB3X/AB3^2 + dD3Z*dD3X/D3^2 + d2BH3XZ/BH3 - d2AB3XZ/AB3 -d2D3XZ/D3) ;
d3Delta3XYY=(x3-r)/D3^3*(DH3-y3^2-3*y3*DH3*dD3Y/D3);
d3Delta3XXY=y3/D3^3*(DH3-(x3-r)^2*(1+3*(DH3/D3)^2));
d3Delta3YYZ=z3/D3^3*(DH3-y3^2-3*y3*DH3*dD3Y/D3);
d3Delta3YZZ=y3/D3^3*(DH3-z3^2*(1+3*(DH3/D3)^2));
d3Delta3XYZ=-(x3-r)*y3*z3/D3^3*(1+3*(DH3/D3)^2);
dHdelta3X=[ d3Delta3XXX,d3Delta3XXY,d3Delta3XXZ ; d3Delta3XXY, d3Delta3XYY,d3Delta3XYZ ;d3Delta3XXZ , d3Delta3XYZ,d3Delta3XZZ] ;
dHdelta3Y=[ d3Delta3XXY,d3Delta3XYY,d3Delta3XYZ ; d3Delta3XYY, d3Delta3YYY,d3Delta3YYZ ;d3Delta3XYZ , d3Delta3YYZ,d3Delta3YZZ] ;
dHdelta3Z=[ d3Delta3XXZ,d3Delta3XYZ,d3Delta3XZZ ; d3Delta3XYZ, d3Delta3YYZ,d3Delta3YZZ ;d3Delta3XZZ , d3Delta3YZZ,d3Delta3ZZZ] ;
d3Delta3= 3*dP3'*Hdelta3*d2P3 + Gdelta3*d3P3 + dP3'*[dHdelta3X*dP3,dHdelta3Y*dP3 , dHdelta3Z*dP3]*dP3 ;
%--------------  les derivees partielles  d3Beta3_
d3Beta3XXX=-2*z3/AB3^4*(1-4*((x3-r)/AB3)^2) ; 
d3Beta3ZZZ=2*(x3-r)/AB3^4*(1-4*(z3/AB3)^2) ; 
d3Beta3XZZ=-d3Beta3XXX;d3Beta1XXZ=-d3Beta3ZZZ ;
dHbeta3X=[d3Beta3XXX , 0 ,d3Beta1XXZ ; 0,0,0;d3Beta1XXZ , 0 , d3Beta3XZZ];
dHbeta3Z=[d3Beta1XXZ , 0 ,d3Beta3XZZ ; 0,0,0;d3Beta3XZZ , 0 , d3Beta3ZZZ];
dHbeta3Y= zeros(3) ;
d3Beta3=3*dP3'*Hbeta3*d2P3 + Gbeta3*d3P3 + dP3'*[dHbeta3X*dP3,dHbeta3Y*dP3, dHbeta3Z*dP3]*dP3 ;
% En fin :
dHalpha3X=dHbeta3X-dHdelta3X ;
dHalpha3Y=dHbeta3Y-dHdelta3Y ;
dHalpha3Z=dHbeta3Z-dHdelta3Z ;
d3Alpha3=3*dP3'*Halpha3*d2P3 + Galpha3*d3P3 + dP3'*[dHalpha3X*dP3,dHalpha3Y*dP3, dHalpha3Z*dP3]*dP3 ;

d3alpha=[ d3Alpha1 ; d3Alpha2 ; d3Alpha3 ];

== matlab function Commande_1_ModeGlissant/RDelta_analityque/MDD/MDD/d2P par Calcule inverse /MCD ==
  data: P output; alpha input; dalpha input; dP output
function [P,dP]= fcn(alpha,dalpha)

% alpha=alpha*pi/180;
% dalpha=dalpha*pi/180;
% d2alpha=d2alpha*pi/180;
alpha1=alpha(1) ;alpha2=alpha(2) ; alpha3=alpha(3) ;
dalpha1=dalpha(1) ;dalpha2=dalpha(2) ; dalpha3=dalpha(3) ;

%% Remarque: une letrre majiscule signifie un point ou un vecteur 
% tandit que un miniscule signifie la norme
%% les constantes
l1 = 0.19992; 
l2 = 0.334; 
r = 0.126; 
phi2 = 2*pi/3;
phi3 = 4*pi/3;
% Fin
%% les points Ci :
OC1=[r+l1*cos(alpha1) ; 0 ; -l1*sin(alpha1) ]; 
OC2=[(r+l1*cos(alpha2))*cos(phi2) ; (r+l1*cos(alpha2))*sin(phi2) ; -l1*sin(alpha2) ]; 
OC3=[(r+l1*cos(alpha3))*cos(phi3) ; (r+l1*cos(alpha3))*sin(phi3) ; -l1*sin(alpha3) ]; 
%% Les veccteurs CiCj :
C1C2=OC2-OC1; C2C3=OC3-OC2 ; C3C1=OC1-OC3;
%% vitesses de point Ci et CiCj:
% dC1= Q1*dAlpha1;
Q1=[-l1*sin(alpha1) ; 0 ; -l1*cos(alpha1)] ; 
Q2=[-l1*sin(alpha2)*cos(phi2) ; -l1*sin(alpha2)*sin(phi2) ; -l1*cos(alpha2)] ;
Q3=[-l1*sin(alpha3)*cos(phi3) ; -l1*sin(alpha3)*sin(phi3) ; -l1*cos(alpha3)] ;
dOC1=Q1*dalpha1 ;
dOC2=Q2*dalpha2 ;
dOC3=Q3*dalpha3 ;
dC1C2=dOC2-dOC1 ; dC2C3=dOC3-dOC2 ; dC3C1=dOC1-dOC3 ;

%% Les longueurs a,b,et c:
a=sqrt(C1C2'*C1C2);
b=sqrt(C2C3'*C2C3);
c=sqrt(C3C1'*C3C1);

%% Calcule de R et s :
p=a+b+c ; % le perimetre
p1=p-2*a ; p2=p-2*b ;  p3=p-2*c ; 
R=a*b*c/sqrt(p*p1*p2*p3); % le Rayon du C1C2C3
s=a*b*c/(2*R); % La surface
V1=C1C2/a; % les vecteures unitaires portes sur les segments
V2=C2C3/b;
V3=C3C1/c;
%% Calcule de n et w:
n=cross(C3C1,C1C2)/s ; % le Vecteur normale
w=sign(-a*a+c*c+b*b)*cross(n,V1) ;
%% les segments  tl=|TK| , ml=|ML| ,lp=|LP|
tl=sqrt(R^2-(a/2)^2);
ml=sqrt(R^2-(b/2)^2);
kl=sqrt(R^2-(c/2)^2);
lp=sqrt(l2^2-R^2) ;
%% les vitess de a,b,et c:
da=V1'*dC1C2;
db=V2'*dC2C3;
dc=V3'*dC3C1;
%% Calcule de dR:
dp=da+db+dc ;
dp1=dp-2*da ; dp2=dp-2*db ; dp3=dp-2*dc ;
dR = ( da/a + db/b + dc/c - 0.5*( dp/p + dp1/p1 + dp2/p2 + dp3/p3 ))*R ;
%dR = ( 1 - 4*R*tl/b/c)*R*da/a + (1-4*R*ml/a/c)*R*db/b + (1-4*R*kl/a/b)*R*dc/c ;
%% Calcule de :
dtl=(R*dR-a*da/4)/tl ;
dlp  = -R*dR/lp ;
ds = (da/a + db/b + dc/c - dR/R)*s ;
dV1=(dC1C2-da*V1)/a ;

dS = cross(dC3C1,C1C2) + cross(C3C1,dC1C2) ;
dn= (dS-ds*n)/s ;
dw=sign(-a*a+c*c+b*b)*(cross(dn,V1) + cross(n,dV1)) ;
% Calcule de P :
OL = (OC1+OC2)/2 + tl*w;
P = OL-lp*n ;
% Calcule de dP :
dOT = (dOC2 + dOC1)/2 ; 
dTL = dtl*w + tl*dw ;
dLP = -dlp*n - lp*dn ; 
dP = dOT + dTL + dLP ;

== matlab function Commande_1_ModeGlissant/Regulateur Mode Glissant/Regulateur ModeGlissant ==
  data: x1 input; U output; x2 input; x3 input; M input; N input; r input; dr input; d2r input; dv input; v output
function [U,v]= fcn(x1,x2,x3,M,N,r,dr,d2r,dv)

%% Mode glissant
% Les Constantes des moteurs ;
Ki =0.119 ; %N-m/A 
b1 = -1.1250e+03 ;
b2 = -99.4718 ;
b3 =833.3333 ;
N=N*Ki ;
%Constantes du Reglage :
l1= 50 ; l2 =80 ;K = 90 ;
Dx1=x1-r ;
dDx1=x2-dr ;
s1 = x2+l1*Dx1-dr ;
v = -N\(-l2*s1-M-l1*dDx1+d2r) ;
s2 = x3 + v ;
U=1/b3*(-K*sign(s2)-b2*x2-b1*x3-dv) ;

== matlab function Commande_1_ModeGlissant/Point de Fonctionnement/Derivee de Tg/Gravite_lineaire ==
  data: Tg output; P input; alpha input; dTg_Theta output; Jinv input
function [Tg,dTg_Theta]= fcn(P,alpha,Jinv)

    alpha1=alpha(1) ;alpha2=alpha(2) ; alpha3=alpha(3) ;
    
%% les constantes:
l1 = 0.19992; 
l2 = 0.334; 
r = 0.126; 
phi2 = 2*pi/3;
phi3 = 4*pi/3;
A2=[cos(phi2) sin(phi2) 0 
     -sin(phi2) cos(phi2) 0
        0            0            1 ]; 
A3=[cos(phi3) sin(phi3) 0
     -sin(phi3) cos(phi3) 0
          0            0          1 ];
g = 9.98 ;
mBras = 0.083660682814532691 ;
mRoue =0.1805;
dBras = 0.058869490365843639 ;
dRoue = 0.0344586;
M2= 2*0.01438 ;
M3 = 0.0416;
shift = 0.0651;
%% Parametres :
    % A) les vecteurs OAi et OBi :
    OA1=[r ; 0 ; 0] ; OA2=[r*cos(phi2) ; r*sin(phi2) ; 0] ; OA3=[r*cos(phi3) ; r*sin(phi3) ; 0] ;
    OC1=[r+l1*cos(alpha1) ; 0 ; -l1*sin(alpha1) ]; 
    OC2=[(r+l1*cos(alpha2))*cos(phi2) ; (r+l1*cos(alpha2))*sin(phi2) ; -l1*sin(alpha2) ]; 
    OC3=[(r+l1*cos(alpha3))*cos(phi3) ; (r+l1*cos(alpha3))*sin(phi3) ; -l1*sin(alpha3) ]; 
    % B) Les vecteurs AiCi :
    A1C1=OC1-OA1 ; A2C2=OC2-OA2 ; A3C3=OC3-OA3 ;
    % Fin

%% ===============-------=====  Calcule de Cgi =====---------====================

% Les vecteurs unitaires portes par les bras paralleles : la nouvelle base
    u1=(P-OC1)/l2 ; u2=(P-OC2)/l2 ; u3=(P-OC3)/l2 ;
    U = [u1 u2 u3] ;

% Les forces aux points Ci ;
     N1=[-dBras*mBras*sin(shift) - dRoue*mRoue*cos(shift) ; 0 ; -dBras*mBras*cos(shift) + dRoue*mRoue*sin(shift)]*g/l1; 
    N2=[0 ;0 ; -M2*g/2] ;
    N=N1+N2;

% les effets totales appliquees a  la nacelle (N4):
    N4 = [0 ; 0 ; -(M3 + M2*3/2)*g] ;

% les composants de N4 sur les bras paralleles = Expression de N4 dans la Nouvelle base U:
    E1 = [1 0 0]; E2 = [0 1 0]; E3 = [0 0 1];
    Z = U\N4 ;
    Z1=(E1*Z)*u1; 
    Z2=(E2*Z)*u2;  
    Z3=(E3*Z)*u3 ;

% les matrices de transformation au plan OXiZi (Bi) :
    B1= [1 0 0; 0 0 0 ; 0 0 1] ;
    B2=B1*A2; B3=B1*A3 ;
% Le couple Cg1 au point de fonc P0:
Cg1 = E2*cross(A1C1,N + B1*Z1);
Cg2 = E2* cross(A2*A2C2,N + B2*Z2)  ;
Cg3 = E2* cross(A3*A3C3, N + B3*Z3) ;
Cg =[Cg1 ;Cg2;Cg3] ;
Tg=Cg/12 ;
%% =========================== Linearisation ================================

% A) la derivee de ACi par rapport au alphai
    dAC1_1=[-l1*sin(alpha1) ; 0 ; -l1*cos(alpha1) ] ; 
    dAC2_2=A2'*[-l1*sin(alpha2); 0 ; -l1*cos(alpha2) ] ;
    dAC3_3=A3'*[-l1*sin(alpha3); 0 ; -l1*cos(alpha3)] ;

% B) les derivees partielles de la matrice U  par rapport au Apha_i
    % les derivees partielles de u1 par rapport au alphai
    du1_1=(Jinv*E1'-dAC1_1)/l2 ; 
    du1_2=(Jinv*E2')/l2 ; 
    du1_3=(Jinv*E3')/l2 ;
    % les derivees partielles de u2 par rapport au alphai
    du2_1=(Jinv*E1')/l2 ; 
    du2_2=(Jinv*E2'-dAC2_2)/l2 ; 
    du2_3=du1_3 ;
    % la derivee partielle de u3 par rapport au alphai
    du3_1=du2_1; 
    du3_2=du1_2; 
    du3_3=(Jinv*E3'-dAC3_3)/l2 ;
    % finalement
    dU_1=[du1_1 , du2_1 , du3_1]; % la derivee partielle de la matrice U par rapport au alpha1
    dU_2=[du1_2 , du2_2 , du3_2]; % la derivee partielle de la matrice U par rapport au alpha2
    dU_3=[du1_3 , du2_3 , du3_3]; % la derivee partielle de la matrice U par rapport au alpha3
    %dU = dU_1*dalpha(1) + dU_2*dalpha(2) +dU_3*dalpha(3) ;

% C) les derivees partielles de Z par rapport au alpha_i
    dZ_1=-U\dU_1*Z ;
    dZ_2=-U\dU_2*Z ;
    dZ_3=-U\dU_3*Z ;
    %dZ=dZ_1*Dalpha(1)+ dZ_2*Dalpha(2) + dZ_3*Dalpha(3) ;

% D) les derivee partilles de Zi par rapport au alpha_i :
    % La derivee de Z1 par rapport au alphai
    dZ1_1 = (E1*dZ_1)*u1+(E1*Z)*du1_1 ;
    dZ1_2 = (E1*dZ_2)*u1+(E1*Z)*du1_2 ;
    dZ1_3 = (E1*dZ_3)*u1+(E1*Z)*du1_3 ;
    % La derivee de Z2 par rapport au alphai
    dZ2_1 = (E2*dZ_1)*u2+(E2*Z)*du2_1 ;
    dZ2_2 = (E2*dZ_2)*u2+(E2*Z)*du2_2 ;
    dZ2_3 = (E2*dZ_3)*u2+(E2*Z)*du2_3 ;
    % La derivee de Z3 par rapport au alphai
    dZ3_1 = (E3*dZ_1)*u3+(E3*Z)*du3_1 ;
    dZ3_2 = (E3*dZ_2)*u3+(E3*Z)*du3_2 ;
    dZ3_3 = (E3*dZ_3)*u3+(E3*Z)*du3_3 ;
    %dZ3=dZ3_1*dalpha(1)+ dZ3_2*dalpha(2) + dZ3_3*dalpha(3) ;

%% E) les derivees partilles de Cgi par rapport au alpha_i :

    % 1) Les derivees partielles de Cg1:
    dCg1_1 = E2* cross(dAC1_1, N + B1*Z1) + E2*cross(A1C1 , B1*dZ1_1) ;
    dCg1_2 = E2*cross(A1C1 , B1*dZ1_2) ;
    dCg1_3 = E2*cross(A1C1 , B1*dZ1_3) ;
    dCg1_alpha = [dCg1_1 , dCg1_2 , dCg1_3] ; % dimension :1*3
    %dCg1= dCg1_1*Dalpha(1) + dCg1_2*Dalpha(2)  + dCg1_3*Dalpha(3) ;
    
    % 2) Les derivees partielles de Cg2:
    dCg2_1 = E2*cross(A2*A2C2 , B2*dZ2_1) ;
    dCg2_2 = E2* cross(A2*dAC2_2, N + B2*Z2) + E2*cross(A2*A2C2 , B2*dZ2_2) ;
    dCg2_3 = E2*cross(A2*A2C2 , B2*dZ2_3) ;
    dCg2_alpha = [dCg2_1 , dCg2_2 , dCg2_3] ;
    %dCg2= dCg2_1*Dalpha(1) + dCg2_2*Dalpha(2)  +dCg2_3*Dalpha(3) ;

    % 3) Les derivees partielles de Cg3:
    dCg3_1 = E2*cross(A3*A3C3 , B3*dZ3_1) ;
    dCg3_2 = E2*cross(A3*A3C3 , B3*dZ3_2) ;
    dCg3_3 = E2*cross(A3*dAC3_3, N + B3*Z3) + E2*cross(A3*A3C3 , B3*dZ3_3) ;
    dCg3_alpha = [dCg3_1 , dCg3_2 , dCg3_3] ;
    %dCg3= dCg3_1*Dalpha(1) + dCg3_2*Dalpha(2)  +dCg3_3*Dalpha(3) ;

dCg_alpha = [dCg1_alpha;dCg2_alpha;dCg3_alpha] ;

%% Les derivees partielles de Tg :
%Theta = alpha*12 ; dTheta = dalpha*12 ; 
dTg_Theta = dCg_alpha/12^2 ; %% RQ :dTg_Theta = dTg_alpha/12
%dTg = dTg_Theta * dTheta ;

== matlab function Commande_1_ModeGlissant/Point de Fonctionnement/Derivee de Tg/Jinv ==
  data: P input; Jinv output
function Jinv= fcn(P)

l1 = 0.19992; 
l2 = 0.334; 
r = 0.126; 
phi2 = 2*pi/3;
phi3 = 4*pi/3;

%% projection de P sur Ri
A2=[cos(phi2) sin(phi2) 0
    -sin(phi2) cos(phi2) 0
    0            0      1 ]; 
A3=[cos(phi3) sin(phi3) 0
    -sin(phi3) cos(phi3) 0
    0            0      1 ];
P2=A2*P; P3=A3*P ;

x1=P(1); y1=P(2) ; z1=P(3) ; %% p1=p
x2=P2(1); y2=P2(2) ; z2=P2(3) ;
x3=P3(1); y3=P3(2) ; z3=P3(3) ;

%% Calcule de ABi et ei :
AB1=sqrt(z1^2+(x1-r)^2);
e1=sqrt(l2^2-y1^2); 
AB2=sqrt(z2^2+(x2-r)^2);
e2=sqrt(l2^2-y2^2);
AB3=sqrt(z3^2+(x3-r)^2);
e3=sqrt(l2^2-y3^2);

%% calcul de alpha1
gama1=acos((AB1^2 + l1^2 - e1^2)/(2*l1*AB1));
gama2=acos((AB2^2 + l1^2 - e2^2)/(2*l1*AB2));
gama3=acos((AB3^2 + l1^2 - e3^2)/(2*l1*AB3));

%% =========== Calcule de  J1  ================
% J1 est defini par : dalpha1= J1*dP
AB1 = sqrt(z1^2+(x1-r)^2);
AH1 = AB1-l1*cos(gama1);
D1=1/(l1*AB1*sin(gama1));
a1 = D1*AH1*(x1-r)/AB1 +  z1/( z1^2 + (x1-r)^2 );
a2 = D1*y1 ;
a3 = D1*AH1*z1/AB1 -(x1-r)/( z1^2 + (x1-r)^2 ) ;
j1= [a1 a2 a3] ;

%% =========== Calcule de  J2  ================
% J2 est defini par : dalpha2 = J2*A2*dP
AB2 = sqrt(z2^2+(x2-r)^2);
AH2 = AB2-l1*cos(gama2);
D2=1/(l1*AB2*sin(gama2));
a4 = D2*AH2*(x2-r)/AB2 + z2/( z2^2 + (x2-r)^2 ) ;
a5 = D2*y2;
a6 = D2*AH2*z2/AB2 -(x2-r)/( z2^2 + (x2-r)^2 );
j2=[a4 a5 a6]*A2;

%%  ========= (dAlpha3)  ================

AB3 = sqrt(z3^2+(x3-r)^2);
AH3 = AB3-l1*cos(gama3);
D3=1/(l1*AB3*sin(gama3));
a7 = D3*AH3*(x3-r)/AB3 + z3/( z3^2 + (x3-r)^2 );
a8 = D3*y3;
a9 = D3*AH3*z3/AB3 -(x3-r)/( z3^2 + (x3-r)^2 ) ;
j3=[ a7 a8 a9]*A3 ;

%% La matrice inverse de J
J=[ j1 ; j2 ; j3 ];
%  dAlpha=J*dp;   
Jinv=eye(3,3) /J;

== matlab function Commande_1_ModeGlissant/RDelta_analityque/MDD/MDD/Gravite_lineaire ==
  data: alpha input; Cg output; P input
function Cg = fcn(alpha,P)

    alpha1=alpha(1) ;alpha2=alpha(2) ; alpha3=alpha(3) ;
    
%% les constantes:
l1 = 0.19992; 
l2 = 0.334; 
r = 0.126; 
phi2 = 2*pi/3;
phi3 = 4*pi/3;
A2=[cos(phi2) sin(phi2) 0 
     -sin(phi2) cos(phi2) 0
        0            0            1 ]; 
A3=[cos(phi3) sin(phi3) 0
     -sin(phi3) cos(phi3) 0
          0            0          1 ];
g = 9.98 ;
mBras = 0.083660682814532691 ;
mRoue =0.1805;
dBras = 0.058869490365843639 ;
dRoue = 0.0344586;
M2= 2*0.01438 ;
M3 = 0.0416;
shift = 0.0651;
%% Parametres :
    % A) les vecteurs OAi et OBi :
    OA1=[r ; 0 ; 0] ; OA2=[r*cos(phi2) ; r*sin(phi2) ; 0] ; OA3=[r*cos(phi3) ; r*sin(phi3) ; 0] ;
    OC1=[r+l1*cos(alpha1) ; 0 ; -l1*sin(alpha1) ]; 
    OC2=[(r+l1*cos(alpha2))*cos(phi2) ; (r+l1*cos(alpha2))*sin(phi2) ; -l1*sin(alpha2) ]; 
    OC3=[(r+l1*cos(alpha3))*cos(phi3) ; (r+l1*cos(alpha3))*sin(phi3) ; -l1*sin(alpha3) ]; 
    % B) Les vecteurs AiCi :
    A1C1=OC1-OA1 ; A2C2=OC2-OA2 ; A3C3=OC3-OA3 ;
    % Fin

%% ===============-------=====  Calcule de Cgi =====---------====================

% Les vecteurs unitaires portes par les bras paralleles : la nouvelle base
    u1=(P-OC1)/l2 ; u2=(P-OC2)/l2 ; u3=(P-OC3)/l2 ;
    U = [u1 u2 u3] ;

% Les forces aux points Ci ;
     N1=[-dBras*mBras*sin(shift) - dRoue*mRoue*cos(shift) ; 0 ; -dBras*mBras*cos(shift) + dRoue*mRoue*sin(shift)]*g/l1; 
    N2=[0 ;0 ; -M2*g/2] ;
    N=N1+N2;

% les effets totales appliquees a  la nacelle (N4):
    N4 = [0 ; 0 ; -(M3 + M2*3/2)*g] ;

% les composants de N4 sur les bras paralleles = Expression de N4 dans la Nouvelle base U:
    E1 = [1 0 0]; E2 = [0 1 0]; E3 = [0 0 1];
    Z = U\N4 ;
    Z1=(E1*Z)*u1; 
    Z2=(E2*Z)*u2;  
    Z3=(E3*Z)*u3 ;

% les matrices de transformation au plan OXiZi (Bi) :
    B1= [1 0 0; 0 0 0 ; 0 0 1] ;
    B2=B1*A2; B3=B1*A3 ;
% Le couple Cg1 au point de fonc P0:
Cg1 = E2*cross(A1C1,N + B1*Z1);
Cg2 = E2* cross(A2*A2C2,N + B2*Z2)  ;
Cg3 = E2* cross(A3*A3C3, N + B3*Z3) ;
Cg =[Cg1 ;Cg2;Cg3] ;

== matlab function Commande_1_ModeGlissant/Point de Fonctionnement/La tension et le Courant au point de fonctionnement ==
  data: U output; T input; dT input; dTheta input; I output
function [U,I]= fcn(T,dT,dTheta)

Ki =0.119 ; %N-m/A 
b1 = -1.1250e+03 ;
b2 = -99.4718 ;
b3 =833.3333 ;

I = T/Ki ;
dI = dT/Ki ;
U = (dI - b2*dTheta - b1*I)/b3 ;
